simulink library "tetherDragForce_ul"  (R2018b)
settings: Solver=VariableStepAuto  StartTime=0.0  StopTime=10.0  RelTol=1e-3
settings Model: Creator=asiddiq2  LastModifiedBy=asiddiq2

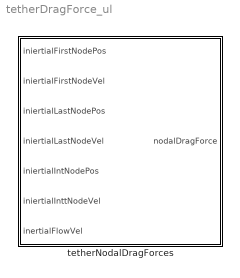
== system tetherDragForce_ul ==
  tetherNodalDragForces : Subsystem  mask{rhoFluid=1, numNode=4, diaTether=1, CdTether=0.5}
      mask prompts: rhoFluid "Fluid density"; numNode "Number of Nodes"; diaTether "Tether diameter"; CdTether "Drag coefficient"
      mask DialogControl Container3 Prompt: Environment
      mask DialogControl ParameterGroupVar Prompt: Tether

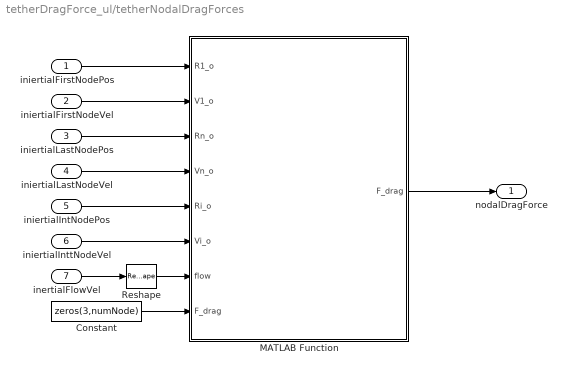
== system tetherDragForce_ul/tetherNodalDragForces ==
  iniertialFirstNodePos : Inport
  iniertialFirstNodeVel : Inport  Port=2
  iniertialLastNodePos : Inport  Port=3
  iniertialLastNodeVel : Inport  Port=4
  iniertialIntNodePos : Inport  Port=5
  iniertialInttNodeVel : Inport  Port=6
  inertialFlowVel : Inport  Port=7
  Constant : Constant  Value=zeros(3,numNode)  VectorParams1D=off
  MATLAB Function : MATLAB Function  TreatAsAtomicUnit=on
  Reshape : Reshape  OutputDimensionality=Column vector (2-D)
  nodalDragForce : Outport
  wires:
  inertialFlowVel/1 -> Reshape/1
  Constant/1 -> MATLAB Function/8("F_drag ")
  Reshape/1 -> MATLAB Function/7(flow)
  iniertialInttNodeVel/1 -> MATLAB Function/6(Vi_o)
  iniertialIntNodePos/1 -> MATLAB Function/5(Ri_o)
  iniertialLastNodeVel/1 -> MATLAB Function/4(Vn_o)
  iniertialLastNodePos/1 -> MATLAB Function/3(Rn_o)
  iniertialFirstNodeVel/1 -> MATLAB Function/2(V1_o)
  iniertialFirstNodePos/1 -> MATLAB Function/1(R1_o)
  MATLAB Function/1(F_drag) -> nodalDragForce/1

== matlab function tetherDragForce_ul/tetherNodalDragForces/MATLAB Function ==
  data: R1_o input; V1_o input; Rn_o input; Vn_o input; Ri_o input; F_drag output; Vi_o input; flow input; F_drag input; CdTether parameter; rhoFluid parameter; numNode parameter; diaTether parameter
function F_drag = fcn(R1_o,V1_o,Rn_o,Vn_o,Ri_o,Vi_o,flow,F_drag,...
    CdTether, rhoFluid, numNode,  diaTether)

if numNode == 2
    Ri_o = [R1_o Rn_o];
    Vi_o = [V1_o Vn_o];
else
    Ri_o = [R1_o Ri_o Rn_o];
    Vi_o = [V1_o Vi_o Vn_o];
end

Ve = zeros(3,numNode-1);
Vrel = zeros(3,numNode-1);
drag_direction = zeros(3,numNode-1);
drag = zeros(3,numNode-1);

qe = zeros(numNode-1,1);
di = zeros(numNode-1,1);
th = zeros(numNode-1,1);
S = zeros(numNode-1,1);

% elemental velocity
for ii = 1:numNode-1
    
    % relative velocity
    Ve(:,ii) = (Vi_o(:,ii) + Vi_o(:,ii+1))/2;                                       % m/s
    Vrel(:,ii) = flow - Ve(:,ii);                                                   % m/s
    Vrel(3,ii) = 0;                                                                 % m/s
    % drag direction
    if norm(Vrel(:,ii)) > 0
        drag_direction(:,ii) = Vrel(:,ii)/norm(Vrel(:,ii));                        % ul
    else
        drag_direction(:,ii) = zeros(3,1);
    end
    
    % dynamic pressure
    qe(ii) = 0.5*rhoFluid*norm(Vrel(:,ii))^2;                                      % N/m^2
    
    % projected area
    di(ii) = norm(Ri_o(:,ii+1)-Ri_o(:,ii));                                         % m
    th(ii) = atan2( (Ri_o(3,ii+1)-Ri_o(3,ii)),norm(Ri_o(1:2,ii+1)-Ri_o(1:2,ii)) );  % rad
    S(ii) = di(ii)*diaTether*sin(th(ii));                                           % m^2
    
    drag(:,ii) = CdTether*qe(ii)*S(ii)*drag_direction(:,ii);
end

% drag force acting on each node'
for ii = 1:numNode
    if ii == 1
        F_drag(:,ii) = drag(:,ii)/2;
    elseif ii> 1 && ii < numNode
        F_drag(:,ii) = (drag(:,ii-1) + drag(:,ii))/2;
    elseif ii == numNode
        F_drag(:,ii) = drag(:,ii-1)/2;
    end
end

end
